simulink model "connecttoUDP_Testing"  (R2025a)
settings: Solver=ode4  StartTime=0.0  StopTime=inf  FixedStep=1/500  RelTol=1e-3  EnableMultiTasking=on
undefined symbols (not defined in the file): HIL, qc_get_step_size
libraries: quarc_library x10
settings Model: Creator=analu  LastModifiedBy=QARM4
settings SolverCC: PositivePriorityOrder=on
settings ModelReferenceCC: EnableRefExpFcnMdlSchedulingChecks=on
settings RTWCC: SystemTargetFile=quarc_win64.tlc  Toolchain=QUARC win64 | nmake (64-bit Windows)  BuildConfiguration=Faster Runs  Description=QUARC Win64 Target Using Toolchain
settings STFCustomTargetCC: SystemTargetFile=quarc_win64.tlc  TargetLangStandard=C99 (ISO)  MultiwordLength=2048.0  DynamicStringBufferSize=256.0  ConcurrentExecutionCompliant=on  UseToolchainInfoCompliant=on
settings GRTTargetCC: ExtMode=on  ExtModeMexFile=quarc_comm  ParMdlRefBuildCompliant=off  CompOptLevelCompliant=off  CombineOutputUpdateFcns=off  MatFileLogging=off  CPPClassGenCompliant=off  GRTInterface=on

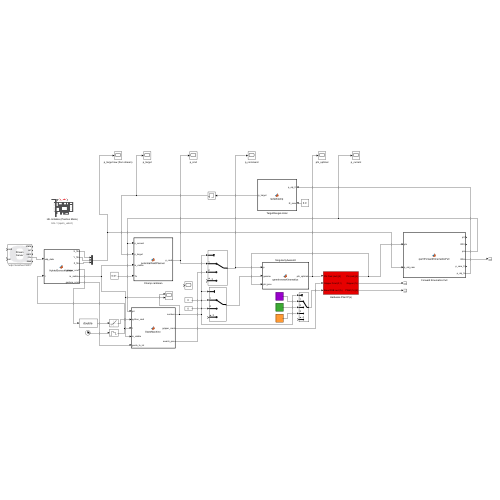
[thumbnail: Simulink's stored preview of the top-level diagram]
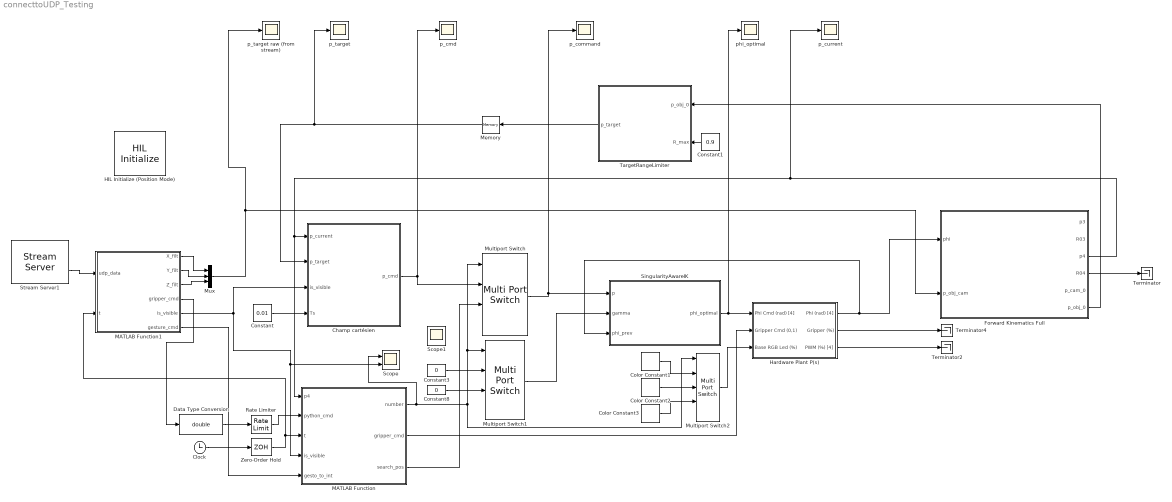
== system connecttoUDP_Testing ==
  Champ cartésien : MATLAB Function  TreatAsAtomicUnit=on
  Clock : Clock
  Color Constant1 : quarc_library/Sources/Signals/Color Constant  color=[0.6 0 0.8]
      settings: SourceProductName=QUARC Targets
  Color Constant2 : quarc_library/Sources/Signals/Color Constant  color=[0.23137 0.66667 0.19608]
      settings: SourceProductName=QUARC Targets
  Color Constant3 : quarc_library/Sources/Signals/Color Constant  color=[1 0.6 0.2]
      settings: SourceProductName=QUARC Targets
  Constant : Constant  Value=0.01
  Constant1 : Constant  Value=0.9
  Constant3 : Constant  Value=0
  Constant8 : Constant  Value=0
  Data Type Conversion : DataTypeConversion  OutMin=0  OutMax=11  OutDataTypeStr=double  SaturateOnIntegerOverflow=off  RndMeth=Floor
  Forward Kinematics Full : MATLAB Function  TreatAsAtomicUnit=on
  HIL Initialize (Position Mode) : quarc_library/Data Acquisition/Generic/Configuration/HIL Initialize  object_name=HIL-1  board_type=qarm_usb  board_number=0  board_options=j0_mode=0;j1_mode=0;j2_mode=0;j3_mode=0;gripper_mode=0;j0_profile_config=0;j0_profile_velocity=1.5708;j0_profile_acceleration=1.0472;j1_profile_config=0;j1_profile_velocity=1.5708;j1_profile_acceleration=1.0472;j2_profile_config=0;j2_profile_velocity=1.5708;j2_profile_acceleration=1.0472;j3_profile_config=0;j3_profile_velocity=1.5708;j3_profile_acceleration=1.0472;  exclusive=off  active=on  hardware_clocks=[0]  clock_modes=[]  initial_clock_frequencies=[]  set_clock_params_at_start=off  set_clock_params_at_switch_in=off  set_clock_frequencies_at_start=off  set_clock_frequencies_at_switch_in=off  analog_input_channels=[5:9]  analog_input_configurations=[]  analog_input_maximums=[]  analog_input_minimums=[]  set_analog_input_params_at_start=off  set_analog_input_params_at_switch_in=off  analog_output_channels=[]  analog_output_maximums=inf  analog_output_minimums=-inf  initial_analog_outputs=[0]  final_analog_outputs=[0]  watchdog_analog_outputs=[]  set_analog_output_params_at_start=off  set_analog_output_params_at_switch_in=off  set_analog_outputs_at_start=off  set_analog_outputs_at_switch_in=off  set_analog_outputs_at_terminate=off  set_analog_outputs_at_switch_out=off  set_analog_outputs_on_watchdog=off  digital_input_channels=[]  digital_output_channels=[]  digital_output_configuration=[]  initial_digital_outputs=[0]  final_digital_outputs=[0]  watchdog_digital_outputs=[0]  set_digital_output_params_at_start=off  set_digital_output_params_at_switch_in=off  set_digital_outputs_at_start=off  set_digital_outputs_at_switch_in=off  set_digital_outputs_at_terminate=off  set_digital_outputs_at_switch_out=off  set_digital_outputs_on_watchdog=off  encoder_channels=[]  quadrature=[]  encoder_filter_frequency=[]  initial_encoder_counts=[]  set_encoder_params_at_start=off  set_encoder_params_at_switch_in=off  set_encoder_counts_at_start=off  set_encoder_counts_at_switch_in=off  pwm_channels=[]  pwm_modes=[]  pwm_frequency=[]  pwm_configuration=[]  pwm_alignment=[]  pwm_polarity=[]  pwm_leading_deadband=[]  pwm_trailing_deadband=[]  initial_pwm_outputs=[]  final_pwm_outputs=[]  watchdog_pwm_outputs=[]  set_pwm_params_at_start=off  set_pwm_params_at_switch_in=off  set_pwm_outputs_at_start=off  set_pwm_outputs_at_switch_in=off  set_pwm_outputs_at_terminate=off  set_pwm_outputs_at_switch_out=off  set_pwm_outputs_on_watchdog=off  other_output_channels=[1000:1004 11000:11003 11005:11007]  initial_other_outputs=[zeros(1,9), ones(1,3)]  final_other_outputs=[zeros(1,9), ones(1,3)]  watchdog_other_outputs=zeros(1,12)  set_other_outputs_at_start=off  set_other_outputs_at_switch_in=off  set_other_outputs_at_terminate=on  set_other_outputs_at_switch_out=off  set_other_outputs_on_watchdog=off
  Hardware Plant P(s) : Subsystem
  MATLAB Function : MATLAB Function  TreatAsAtomicUnit=on
  MATLAB Function1 : MATLAB Function  TreatAsAtomicUnit=on
  Memory : Memory  InitialCondition=[0 ,0.5 ,0.5]
  Multiport Switch : MultiPortSwitch  SaturateOnIntegerOverflow=off  InputSameDT=off
  Multiport Switch1 : MultiPortSwitch  SaturateOnIntegerOverflow=off  InputSameDT=off
  Multiport Switch2 : MultiPortSwitch  Inputs=4  SaturateOnIntegerOverflow=off  InputSameDT=off
  Mux : Mux  Inputs=3
  Rate Limiter : RateLimiter  SampleTimeMode=inherited
  Scope : Scope  NumInputPorts=2
      settings: ActiveDisplayYMinimum=-0.24999999999999994  ActiveDisplayYMaximum=2.25  DataLoggingVariableName=ScopeData8
  Scope1 : Scope
      settings: DataLoggingVariableName=ScopeData9
  SingularityAwareIK : MATLAB Function  TreatAsAtomicUnit=on
  Stream Server1 : quarc_library/Communications/Basic/Stream Server  uri_source=Specify via dialog (do not evaluate)  uri=udp://localhost:5005  send_buffer_size=1460  receive_buffer_size=1460  byte_order=little endian (Intel - LSB first)  optimization=Minimum latency  send_options=Send all data  receive_options=Receive all data  default_value=[0,0,0,0,0,0,0,0]  sample_time=qc_get_step_size  active=off  implementation=Use blocking I/O in a separate thread  send_fifo_size=1000  receive_fifo_size=1000  send_priority=0  receive_priority=0  send_dimensions=off  receive_dimensions=off  max_dimensions=-1  data_type=single  type_expr=BusObject
      settings: AttributesFormatString="\"udp://localhost:5005\""
  TargetRangeLimiter : MATLAB Function  TreatAsAtomicUnit=on
  Terminator : Terminator
  Terminator2 : Terminator
  Terminator4 : Terminator
  Zero-Order Hold : ZeroOrderHold  SampleTime=-1
  p_cmd : Scope
      settings: ActiveDisplayYMinimum=-0.053062727209180587  ActiveDisplayYMaximum=0.31034032395109534
  p_command : Scope
      settings: ActiveDisplayYMinimum=-0.053062727209180587  ActiveDisplayYMaximum=0.31034032395109534  DataLoggingVariableName=ScopeData3
  p_current : Scope
      settings: ActiveDisplayYMinimum=-0.053062727209180587  ActiveDisplayYMaximum=0.31034032395109534  DataLoggingVariableName=ScopeData6
  p_target : Scope
      settings: ActiveDisplayYMinimum=-0.053062727209180587  ActiveDisplayYMaximum=0.31034032395109534  DataLoggingVariableName=ScopeData7
  p_target raw (from stream) : Scope
      settings: ActiveDisplayYMinimum=-0.053062727209180587  ActiveDisplayYMaximum=0.31034032395109534  DataLoggingVariableName=ScopeData2
  phi_optimal : Scope
      settings: ActiveDisplayYMinimum=-0.053062727209180587  ActiveDisplayYMaximum=0.31034032395109534
  wires:
  Stream Server1/4 -> MATLAB Function1/1(udp_data)
  SingularityAwareIK/1(phi_optimal) -> phi_optimal/1, Hardware Plant P(s)/1(Phi Cmd (rad) [4])
  Constant/1 -> Champ cartésien/4(Ts)
  Hardware Plant P(s)/1(Phi (rad) [4]) -> SingularityAwareIK/3(phi_prev), Forward Kinematics Full/1(phi)
  Hardware Plant P(s)/2(Gripper (%)) -> Terminator4/1
  Hardware Plant P(s)/3(PWM (%) [4]) -> Terminator2/1
  Multiport Switch/1 -> p_command/1, SingularityAwareIK/1(p)
  Champ cartésien/1(p_cmd) -> p_cmd/1, Multiport Switch/2
  MATLAB Function/3(search_pos) -> Multiport Switch/3
  MATLAB Function/2(gripper_cmd) -> Hardware Plant P(s)/2(Gripper Cmd (0,1))
  Multiport Switch2/1 -> Hardware Plant P(s)/3(Base RGB Led (%))
  Multiport Switch1/1 -> SingularityAwareIK/2(gamma)
  MATLAB Function/1(number) -> Scope/1, Multiport Switch2/1, Multiport Switch/1, Multiport Switch1/1
  Constant3/1 -> Multiport Switch1/2
  Constant8/1 -> Multiport Switch1/3
  Zero-Order Hold/1 -> MATLAB Function1/2(t), MATLAB Function/3(t)
  Clock/1 -> Zero-Order Hold/1
  Rate Limiter/1 -> MATLAB Function/2(python_cmd)
  Data Type Conversion/1 -> Rate Limiter/1
  Forward Kinematics Full/3(p4) -> p_current/1, MATLAB Function/1(p4), Champ cartésien/1(p_current)
  Forward Kinematics Full/4(R04) -> Terminator/1
  Forward Kinematics Full/6(p_obj_0) -> TargetRangeLimiter/1(p_obj_0)
  TargetRangeLimiter/1(p_target) -> Memory/1
  Color Constant2/1 -> Multiport Switch2/3
  Color Constant1/1 -> Multiport Switch2/2
  Color Constant3/1 -> Multiport Switch2/4
  Constant1/1 -> TargetRangeLimiter/2(R_max)
  Memory/1 -> p_target/1, Champ cartésien/2(p_target)
  MATLAB Function1/5(is_visible) -> Scope/2, MATLAB Function/4(is_visible), Champ cartésien/3(is_visible)
  Mux/1 -> p_target raw (from stream)/1, Forward Kinematics Full/2(p_obj_cam)
  MATLAB Function1/1(X_filt) -> Mux/1
  MATLAB Function1/2(Y_filt) -> Mux/2
  MATLAB Function1/3(Z_filt) -> Mux/3
  MATLAB Function1/4(gripper_cmd) -> Data Type Conversion/1
  MATLAB Function1/6(gesture_cmd) -> MATLAB Function/5(gesto_to_int)

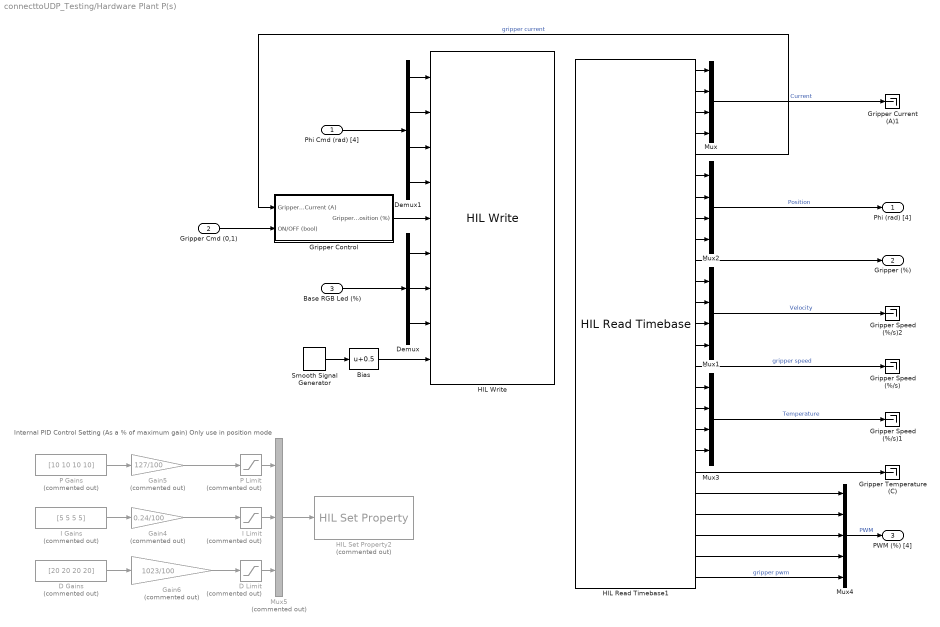
== system connecttoUDP_Testing/Hardware Plant P(s) ==
  note: Internal PID Control Setting (As a % of maximum gain)
      | Only use in position mode
  Phi Cmd (rad) [4] : Inport
  Gripper Cmd (0,1) : Inport  Port=2
  Base RGB Led (%) : Inport  Port=3
  Bias : Bias  Bias=0.5  SaturateOnIntegerOverflow=off
  D Gains : Constant  Commented=on  Value=[20 20 20 20]
  D Limit : Saturate  Commented=on  UpperLimit=[1023 1023 1023 1023]  LowerLimit=[0 0 0 0]
  Demux : Demux  Outputs=3
  Demux1 : Demux
  Gain4 : Gain  Commented=on  Gain=0.24/100
  Gain5 : Gain  Commented=on  Gain=127/100
  Gain6 : Gain  Commented=on  Gain=1023/100
  Gripper Control : Subsystem
  Gripper Current (A)1 : Terminator
  Gripper Speed (%/s) : Terminator
  Gripper Speed (%/s)1 : Terminator
  Gripper Speed (%/s)2 : Terminator
  Gripper Temperature (C) : Terminator
  HIL Read Timebase1 : quarc_library/Data Acquisition/Generic/Timebases/HIL Read Timebase  object_name=HIL-1  clock=0  analog_channels=[5:9]  encoder_channels=[]  digital_channels=[]  other_channels=[1000:1004 3000:3004 10000:10004 11000:11004]  active=on  vector_output=off  data_type_mode=Inherit via back propagation  encoder_data_type=double  digital_data_type=boolean  overflow_mode=Error on overflow  samples_in_buffer=max(ceil(1/qc_get_step_size), 1)
  HIL Set Property2 : quarc_library/Data Acquisition/Generic/Configuration/HIL Set Property  Commented=on  object_name=unassigned  property_type=2  property_codes=[128:131 133:136 138:141]  property_source=2  property_value_num=0  set_at_start=on  sample_time=-1  active=off
      settings: AttributesFormatString=(%<object_name>)  SourceProductName=QUARC Targets
  HIL Write : quarc_library/Data Acquisition/Generic/Immediate I//O/HIL Write  object_name=HIL-1  analog_channels=[]  pwm_channels=[]  digital_channels=[]  other_channels=[1000:1004 11005:11008]  sample_time=-1  active=on  vector_input=off
  I Gains : Constant  Commented=on  Value=[5 5 5 5]
  I Limit : Saturate  Commented=on  UpperLimit=[0.24 0.24 0.24 0.24]  LowerLimit=[0 0 0 0]
  Mux{,1..3} (4 alike) : Mux
  Mux4 : Mux  Inputs=5
  Mux5 : Mux  Commented=on  Inputs=3
  P Gains : Constant  Commented=on  Value=[10 10 10 10]
  P Limit : Saturate  Commented=on  UpperLimit=[127 127 127 127]  LowerLimit=[0 0 0 0]
  Smooth Signal Generator : quarc_library/Sources/Signals/Smooth Signal Generator  signal_type=Sine  source=Internal (dialog parameters)  amplitude=0.5  frequency=60/72  initial_phase=0  sample_time=qc_get_step_size  output_cos=off
      settings: SourceProductName=QUARC Targets
  Phi (rad) [4] : Outport  VectorParamsAs1DForOutWhenUnconnected=off
  Gripper (%) : Outport  Port=2  VectorParamsAs1DForOutWhenUnconnected=off
  PWM (%) [4] : Outport  Port=3  VectorParamsAs1DForOutWhenUnconnected=off
  wires:
  HIL Read Timebase1/10 -> Gripper (%)/1
  Mux4/1 -> PWM (%) [4]/1  "PWM"
  HIL Read Timebase1/25 -> Mux4/5  "gripper pwm"
  HIL Read Timebase1/24 -> Mux4/4
  HIL Read Timebase1/23 -> Mux4/3
  HIL Read Timebase1/22 -> Mux4/2
  HIL Read Timebase1/21 -> Mux4/1
  Mux2/1 -> Phi (rad) [4]/1  "Position"
  Phi Cmd (rad) [4]/1 -> Demux1/1
  Demux1/4 -> HIL Write/4
  Demux1/3 -> HIL Write/3
  Demux1/2 -> HIL Write/2
  Demux1/1 -> HIL Write/1
  Base RGB Led (%)/1 -> Demux/1
  Mux3/1 -> Gripper Speed (%/s)1/1  "Temperature"
  Mux1/1 -> Gripper Speed (%/s)2/1  "Velocity"
  Mux/1 -> Gripper Current (A)1/1  "Current"
  HIL Read Timebase1/20 -> Gripper Temperature (C)/1
  HIL Read Timebase1/1 -> Mux/1
  HIL Read Timebase1/2 -> Mux/2
  HIL Read Timebase1/13 -> Mux1/3
  Demux/2 -> HIL Write/7
  HIL Read Timebase1/19 -> Mux3/4
  Demux/1 -> HIL Write/6
  HIL Read Timebase1/11 -> Mux1/1
  HIL Read Timebase1/16 -> Mux3/1
  HIL Read Timebase1/17 -> Mux3/2
  HIL Read Timebase1/3 -> Mux/3
  Demux/3 -> HIL Write/8
  HIL Read Timebase1/15 -> Gripper Speed (%/s)/1  "gripper speed"
  HIL Read Timebase1/5 -> Gripper Control/1(Gripper Current (A))  "gripper current"
  HIL Read Timebase1/7 -> Mux2/2
  HIL Read Timebase1/4 -> Mux/4
  HIL Read Timebase1/12 -> Mux1/2
  HIL Read Timebase1/8 -> Mux2/3
  HIL Read Timebase1/18 -> Mux3/3
  HIL Read Timebase1/6 -> Mux2/1
  HIL Read Timebase1/9 -> Mux2/4
  HIL Read Timebase1/14 -> Mux1/4
  Gripper Control/1(Gripper Position (%)) -> HIL Write/5
  Gripper Cmd (0,1)/1 -> Gripper Control/2(ON/OFF (bool))
  Smooth Signal Generator/1 -> Bias/1
  Bias/1 -> HIL Write/9
  I Limit/1 -> Mux5/2
  Gain5/1 -> P Limit/1
  D Limit/1 -> Mux5/3
  Mux5/1 -> HIL Set Property2/1
  I Gains/1 -> Gain4/1
  P Gains/1 -> Gain5/1
  D Gains/1 -> Gain6/1
  P Limit/1 -> Mux5/1
  Gain6/1 -> D Limit/1
  Gain4/1 -> I Limit/1

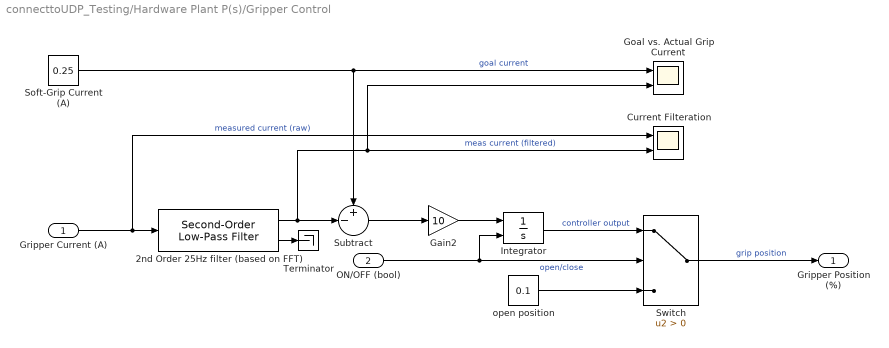
== system connecttoUDP_Testing/Hardware Plant P(s)/Gripper Control ==
  Gripper Current (A) : Inport
  ON/OFF (bool) : Inport  Port=2
  2nd Order 25Hz filter (based on FFT) : quarc_library/Continuous/Second-Order Low-Pass Filter  params_source=Internal (dialog parameters)  input_width=25*2*pi  input_zeta=1  input_init=0
  Current Filteration : Scope  NumInputPorts=2
      settings: ActiveDisplayYMinimum=-0.01447  ActiveDisplayYMaximum=0.62651  DataLoggingVariableName=ScopeData5
  Gain2 : Gain  Gain=10
  Goal vs. Actual Grip Current : Scope  NumInputPorts=2
      settings: ActiveDisplayYMinimum=0.00229  ActiveDisplayYMaximum=0.27702  DataLoggingVariableName=ScopeData4
  Integrator : Integrator  ExternalReset=either  InitialCondition=0.1  LimitOutput=on  UpperSaturationLimit=0.9  LowerSaturationLimit=0.1
  Soft-Grip Current (A) : Constant  Value=0.25
  Subtract : Sum  Inputs=+-|
  Switch : Switch  Criteria=u2 > Threshold  SaturateOnIntegerOverflow=off  InputSameDT=off
  Terminator : Terminator
  open position : Constant  Value=0.1
  Gripper Position (%) : Outport  VectorParamsAs1DForOutWhenUnconnected=off
  wires:
  Gripper Current (A)/1 -> 2nd Order 25Hz filter (based on FFT)/1, Current Filteration/1  "measured current (raw)"
  ON/OFF (bool)/1 -> Switch/2, Integrator/2  "open/close"
  open position/1 -> Switch/3
  Switch/1 -> Gripper Position (%)/1  "grip position"
  Soft-Grip Current (A)/1 -> Subtract/1, Goal vs. Actual Grip Current/1  "goal current"
  2nd Order 25Hz filter (based on FFT)/1 -> Subtract/2, Current Filteration/2, Goal vs. Actual Grip Current/2  "meas current (filtered)"
  Subtract/1 -> Gain2/1
  Integrator/1 -> Switch/1  "controller output"
  Gain2/1 -> Integrator/1
  2nd Order 25Hz filter (based on FFT)/2 -> Terminator/1

== matlab function connecttoUDP_Testing/TargetRangeLimiter ==
  data: p_obj_0 input size=3; p_target output size=3; R_max input
function p_target = radialClamp(p_obj_0, R_max)

eps_val = 1e-6;

norm_p = norm(p_obj_0);

if norm_p > R_max
    p_target = R_max * (p_obj_0 / (norm_p + eps_val));
else
    p_target = p_obj_0;
end

end

== matlab function connecttoUDP_Testing/Champ cartésien ==
  data: p_current input; p_cmd output; p_target input; is_visible input; Ts input
function p_cmd = potentialFieldPlanner(p_current, p_target, is_visible, Ts)
% p_current : [3x1]
% p_target   : [3x1]
% is_visible: 0/1
% Ts        : pas de temps

%% Paramètres
k_att = 2.0;       % gain attractif
k_rep = 0.05;      % gain répulsif cylindre
v_max = 0.25;      % vitesse cartésienne max [m/s]

d0 = 0.15;         % rayon d'influence du cylindre
eps_norm = 1e-6;   % protection division par zéro

%% Si cible non visible : on garde la position actuelle
if is_visible == 0
    p_cmd = p_current;
    return;
end

%% --- Champ attractif ---
e = p_target - p_current;
F_att = k_att * e;

%% --- Champ répulsif cylindre autour de la base ---
x = p_current(1);
y = p_current(2);
d = sqrt(x^2 + y^2);

F_rep = [0;0;0];

if d < d0 && d > eps_norm
    n = [x; y; 0] / (d + eps_norm);
    F_rep = k_rep * (1/d - 1/d0) * (1/(d^2 + eps_norm)) * n;
end

%% --- Champ total ---
F = F_att + F_rep;

%% --- Saturation smooth ---
F_norm = norm(F);

if F_norm > eps_norm
    v_cmd = v_max * tanh(F_norm / v_max) * (F / F_norm);
else
    v_cmd = [0;0;0];
end

%% --- Pas d'Euler ---
p_cmd = p_current + Ts * v_cmd;

end

== matlab function connecttoUDP_Testing/Forward Kinematics Full ==
  data: p3 output; R03 output; phi input; p4 output; R04 output; p_obj_cam input; p_cam_0 output; p_obj_0 output
function [p3, R03, p4, R04, p_cam_0, p_obj_0] = qarmForwardKinematicsFull(phi, p_obj_cam)
%% QARM Forward Kinematics Full
% INPUTS:
%   phi       : angles articulaires QArm [4x1]
%   p_obj_cam : position objet dans le repère caméra [3x1]
%               (mettre [0;0;0] si non utilisée)
%
% OUTPUTS:
%   p3      : position frame {3} dans {0}
%   R03     : rotation frame {3} dans {0}
%   p4      : position effecteur frame {4} dans {0}
%   R04     : rotation effecteur frame {4} dans {0}
%   p_cam_0 : position caméra dans {0}
%   p_obj_0 : position objet dans {0}

%% Paramètres du manipulateur
L1 = 0.1400;
L2 = 0.3500;
L3 = 0.0500;
L4 = 0.2500;
L5 = 0.1500;

%% Paramètres alternatifs
l1 = L1;
l2 = sqrt(L2^2 + L3^2);
l3 = L4 + L5;
beta = atan(L3/L2);

%% Conversion phi -> theta
theta = phi;
theta(1) = phi(1);
theta(2) = phi(2) + beta - pi/2;
theta(3) = phi(3) - beta;
theta(4) = phi(4);

%% Matrices homogènes
T01 = quanser_arm_DH(  0, -pi/2, l1, theta(1) );
T12 = quanser_arm_DH( l2,     0,  0, theta(2) );
T23 = quanser_arm_DH(  0, -pi/2,  0, theta(3) );
T34 = quanser_arm_DH(  0,     0, l3, theta(4) );

T02 = T01*T12;
T03 = T02*T23;
T04 = T03*T34;

%% Sorties principales
p3  = T03(1:3,4);
R03 = T03(1:3,1:3);

p4  = T04(1:3,4);
R04 = T04(1:3,1:3);

%% Caméra
d_tilde = 0.3;                 % distance entre P03 et la caméra
p_cam_3 = [0;0;d_tilde];

% Choisir UNE SEULE orientation caméra
R_cam_3 = [ 0 -1  0;
            1  0  0;
            0  0  1 ];

p_cam_0 = p3 + R03 * p_cam_3;
R_cam_0 = R03 * R_cam_3;

%% Objet
if nargin < 2
    p_obj_cam = [0;0;0];
end

p_obj_0 = p_cam_0 + R_cam_0 * p_obj_cam;

end

function T = quanser_arm_DH(a, alpha, d, theta)

T_R_z = [cos(theta) -sin(theta) 0 0;
         sin(theta)  cos(theta) 0 0;
                  0           0 1 0;
                  0           0 0 1];

T_T_z = [1 0 0 0;
         0 1 0 0;
         0 0 1 d;
         0 0 0 1];

T_T_x = [1 0 0 a;
         0 1 0 0;
         0 0 1 0;
         0 0 0 1];

T_R_x = [1          0           0 0;
         0 cos(alpha) -sin(alpha) 0;
         0 sin(alpha)  cos(alpha) 0;
         0          0           0 1];

T = T_R_z * T_T_z * T_T_x * T_R_x;

end

== matlab function connecttoUDP_Testing/SingularityAwareIK ==
  data: p input; gamma input; phi_optimal output; phi_prev input
function phi_optimal = qarmInverseKinematics(p, gamma, phi_prev)
%% QARM Inverse Kinematics with singularity avoidance
% Gère :
% 1) singularité "effecteur au-dessus de la base" via exclusion cylindrique
% 2) singularité de l'articulation 3 : theta3 = +/- 90 deg
%
% INPUTS:
%   p        : position [x;y;z] en m
%   gamma    : rotation poignet (rad)
%   phi_prev : configuration précédente [4x1] en rad
%
% OUTPUT:
%   phi_optimal : configuration atteignable [4x1] rad

%% Paramètres du manipulateur
L1 = 0.1400; 
L2 = 0.3500; 
L3 = 0.0500; 
L4 = 0.2500; 
L5 = 0.1500;

beta = atan(L3/L2);

lambda1 = L1;
lambda2 = sqrt(L2^2 + L3^2);
lambda3 = L4 + L5;

%% Paramètres d'évitement des singularités A ADAPTER PAS ENCORE DE TEST FAIT SUR ROBOT 
R_MIN = 0.08;                 % rayon mini du cylindre d'exclusion (m)
EPS_DEN = 1e-6;               % protection divisions
EPS_COST = 1e-4;              % protection coût singularité

W_CONT = 1.0;                 % poids continuité avec phi_prev
W_SING_THETA3 = 0.25;         % poids singularité theta3 = +/- pi/2
W_LIMIT = 0.05;               % petit poids pour éloigner des butées

%% --- 1) Exclusion cylindrique autour de la base ---
% On évite une zone cylindrique autour de la base (le bras se bloque quand
% il y entre).
% Ici, on régularise directement la cible cartésienne.
p_reg = p;
r = hypot(p(1), p(2));

if r < R_MIN
    if r > EPS_DEN
        p_reg(1) = p(1) * R_MIN / r;
        p_reg(2) = p(2) * R_MIN / r;
    else
        % Si on est exactement sur l'axe, on prend la direction de la base précédente
        base_dir = phi_prev(1);
        p_reg(1) = R_MIN * cos(base_dir);
        p_reg(2) = R_MIN * sin(base_dir);
    end
end

%% Initialisation
theta = zeros(4,4);
phi   = zeros(4,4);

%% --- Calcul theta2 / theta3 ---
A = lambda2; 
C = -lambda3; 
H = lambda1 - p_reg(3);

D1 = -hypot(p_reg(1), p_reg(2)); 
D2 =  hypot(p_reg(1), p_reg(2));

F1 = (D1^2 + H^2 - A^2 - C^2)/(2*A);
F2 = (D2^2 + H^2 - A^2 - C^2)/(2*A);

% Si racine négative, saturation
if C^2 - F1^2 < 0
    warning('Position non atteignable pour solution 1/2 : saturation');
    theta(3,1) = sign(C)*pi/2;
    theta(3,2) = sign(C)*pi/2;
else
    theta(3,1) = 2*atan2(C + sqrt(C^2 - F1^2), F1);
    theta(3,2) = 2*atan2(C - sqrt(C^2 - F1^2), F1);
end

if C^2 - F2^2 < 0
    warning('Position non atteignable pour solution 3/4 : saturation');
    theta(3,3) = sign(C)*pi/2;
    theta(3,4) = sign(C)*pi/2;
else
    theta(3,3) = 2*atan2(C + sqrt(C^2 - F2^2), F2);
    theta(3,4) = 2*atan2(C - sqrt(C^2 - F2^2), F2);
end

%% --- Calcul theta2 ---
for i = 1:4
    D = D1; 
    if i > 2
        D = D2; 
    end

    M = A + C*sin(theta(3,i));
    N = -C*cos(theta(3,i));

    if abs(M) < EPS_DEN
        M = sign_nonzero(M) * EPS_DEN;
    end

    cos_term = (D*M + H*N)/(M^2 + N^2);
    sin_term = (H - N*cos_term)/M;
    theta(2,i) = atan2(sin_term, cos_term);
end

%% --- Calcul theta1 ---
for i = 1:4
    denom = lambda2*cos(theta(2,i)) - lambda3*sin(theta(2,i)+theta(3,i));
    if abs(denom) < EPS_DEN
        denom = sign_nonzero(denom) * EPS_DEN;
    end
    theta(1,i) = atan2(p_reg(2)/denom, p_reg(1)/denom);
end

%% --- Remap vers angles QARM ---
phi(1,:) = theta(1,:);
phi(2,:) = theta(2,:) - beta + pi/2;
phi(3,:) = theta(3,:) + beta;
phi(4,:) = gamma;

phi = wrapToPiLocal(phi);

%% --- Saturation des limites ---
for i = 1:4
    phi(:,i) = saturate_joint_limits(phi(:,i));
end

%% --- Choix de la meilleure solution avec pénalisation singularités ---
phi_optimal = phi(:,1);
best_cost = candidate_cost(phi(:,1), theta(:,1), phi_prev, R_MIN, r, W_CONT, W_SING_THETA3, W_LIMIT, EPS_COST);

for i = 2:4
    current_cost = candidate_cost(phi(:,i), theta(:,i), phi_prev, R_MIN, r, W_CONT, W_SING_THETA3, W_LIMIT, EPS_COST);
    if isnan(current_cost)
        continue;
    end
    if current_cost < best_cost
        phi_optimal = phi(:,i);
        best_cost = current_cost;
    end
end

if any(isnan(phi_optimal))
    warning('NaN détecté dans phi_optimal, retour à phi_prev');
    phi_optimal = phi_prev;
end

end

%% ===================== COST FUNCTION =====================
function J = candidate_cost(phi_i, theta_i, phi_prev, R_MIN, r_raw, W_CONT, W_SING_THETA3, W_LIMIT, EPS_COST)

    % 1) Continuité avec la configuration précédente
    dphi = wrapToPiLocal(phi_i - phi_prev);
    J_cont = norm(dphi);

    % 2) Pénalisation singularité theta3 = +/- 90 deg
    % Rapport : singularité quand theta3 = +/- pi/2
    d1 = abs(wrapToPiLocal(theta_i(3) - pi/2));
    d2 = abs(wrapToPiLocal(theta_i(3) + pi/2));
    J_sing_theta3 = 1/(d1^2 + EPS_COST) + 1/(d2^2 + EPS_COST);

    % 3) Petite pénalisation si on est près des butées
    J_limits = joint_limit_barrier(phi_i, EPS_COST);

    % 4) Pénalisation brute si la cible originale était trop près de l'axe base
    % (même si régularisée ensuite)
    if r_raw < R_MIN
        J_base = 1 + 10*(R_MIN - r_raw)^2;
    else
        J_base = 0;
    end

    J = W_CONT * J_cont + ...
        W_SING_THETA3 * J_sing_theta3 + ...
        W_LIMIT * J_limits + ...
        J_base;
end

%% ===================== JOINT LIMITS =====================
function phi_sat = saturate_joint_limits(phi)
% C'est les mêmes limites qu'avant mais ça peut être intéressant à régler 
limits = [
    -170  170;
    -80    80;
    -95    75;
    -160  160
] * pi/180;

phi_sat = phi;
for i = 1:4
    if phi(i) < limits(i,1)
        phi_sat(i) = limits(i,1);
    end
    if phi(i) > limits(i,2)
        phi_sat(i) = limits(i,2);
    end
end
end

function J = joint_limit_barrier(phi, eps_cost)
limits = [
    -170  170;
    -80    80;
    -95    75;
    -160  160
] * pi/180;

J = 0;
for k = 1:4
    dmin = abs(phi(k) - limits(k,1));
    dmax = abs(limits(k,2) - phi(k));
    J = J + 1/(dmin^2 + eps_cost) + 1/(dmax^2 + eps_cost);
end
end

%% ===================== HELPERS =====================
function y = wrapToPiLocal(x)
y = mod(x + pi, 2*pi) - pi;
end

function s = sign_nonzero(x)
if x >= 0
    s = 1;
else
    s = -1;
end
end

== matlab function connecttoUDP_Testing/MATLAB Function1 ==
  data: udp_data input size=[8 1]; X_filt output; t input size=1; Y_filt output; Z_filt output; gripper_cmd output; is_visible output; gesture_cmd output size=1
function [X_filt, Y_filt, Z_filt, gripper_cmd, is_visible, gesture_cmd] = HybridSensorKalman(udp_data, t)
    % udp_data is a 7x1 vector from Python: 
    % [SensX, SensY, SensZ, PinhX, PinhY, PinhZ, FoundFlag]
    
    % Define the variables that will remember their values between Simulink steps
    persistent x_est P kf_initialized t_grip_start

    % Initialize the Kalman Filter
    if isempty(kf_initialized)
        x_est = [0.2; 0.0; 0.3]; % Initial guess (Safe home position)
        P = eye(3) * 1.0;        % Initial uncertainty
        kf_initialized = true;
        t_grip_start = -1;       % Timer for gripper delay
    end

    % 1. Unpack UDP data and force double precision
    z_sens = double(udp_data(1:3));
    z_pinh = double(udp_data(4:6));
    found_flag = double(udp_data(7));
    gesture_cmd = double(udp_data(8));

    is_visible = found_flag;
    
    % Kalman tuning parameters (to be adjusted through trial and error)
    Q = eye(3) * 0.001; % Process Noise
    R_val = 0.05;       % Measurement Noise

    % 2. Constant Position Kalman Prediction
    x_est = x_est; 
    P = P + Q;

    % 3. Kalman Update (Sensor Fusion)
    if found_flag == 1
        % Determine depth
        depth = z_sens(3);
        if depth == 0 % Blind sensor scenario
            depth = z_pinh(3);
        end
        
        % Dynamic Confidence (Soft Switch)
        if depth < 0.25
            % Very close: Trust Pinhole 100%, Sensor 0%
            w_sens = 0.0; 
            w_pinh = 1.0;
        elseif depth > 0.35
            % Far away: Trust Sensor 100%, Pinhole 0%
            w_sens = 1.0; 
            w_pinh = 0.0;
        else
            % Transition Zone (25cm to 35cm): Cross-fade the signals
            w_sens = (depth - 0.25) / 0.10; 
            w_pinh = 1.0 - w_sens;
        end
        
        % Fused depth estimation
        z_fused = (w_sens * z_sens) + (w_pinh * z_pinh);
        
        % Calculate Kalman Gain
        R = eye(3) * R_val;
        K = P / (P + R);
        
        % Apply the measurement correction
        x_est = x_est + K * (z_fused - x_est);
        P = (eye(3) - K) * P;
    end

    % 4. Output filtered coordinates
    X_filt = x_est(1);
    Y_filt = x_est(2);
    Z_filt = x_est(3);

    % 5. Gripper Delay Logic
    gripper_cmd = 0;
    
    % Calculate distance from arm base (assuming base is 0,0,0)
    dist_to_target = norm(x_est); 

    if found_flag == 1 && dist_to_target <= 0.18 % COMMIT_DISTANCE variable
        if t_grip_start == -1
            t_grip_start = t; % Start timer
        elseif (t - t_grip_start) >= 0.75 % GRIP_DELAY variable
            gripper_cmd = 1; % Trigger grip
        end
    else
        t_grip_start = -1; % Reset timer if it moves away
    end
end

== matlab function connecttoUDP_Testing/MATLAB Function ==
  data: number output; p4 input; python_cmd input; t input; is_visible input; gripper_cmd output; search_pos output; gesto_to_int input
function [number, gripper_cmd, search_pos] = StateMachine(p4, python_cmd, t, is_visible, gesto_to_int)    
    
    persistent state
    persistent t_travel
    persistent t_visible
    persistent t_lost
    persistent t_gesture
    persistent current_y

    if isempty(state)
        state = 2; % 0 = Hunting the ball down, 1 = Going back to goal, 2 = Returning home and search
        t_travel = -1; % Putting a negative time stops the timer, used to find the travel time in each state mode
        t_visible = -1;
        t_lost = -1;
        t_gesture = -1;
        current_y = 0;
    end
    
    % Default safe position to output when not in State 2
    search_pos = [0.25; 0; 0.50];

    % --- Machine State Logic ---
    switch state
        
        case 0 % STATE 0: HUNTING THE BALL
            number = 1; % Connected on port 1 (xyz_mean)
            gripper_cmd = python_cmd; % The claw follows the camera
            
            % 1. CHECK IF BALL WAS CAUGHT
            if python_cmd == 1
                state = 3; 
                t_lost = -1; % Reset lost timer just in case
            end
            
            % 2. WATCHDOG TIMER: IF BALL IS LOST
            % If the camera goes blind, start the stopwatch before aborting
            if is_visible == 0
                if t_lost == -1
                    t_lost = t; % Start the lost stopwatch
                elseif (t - t_lost) >= 2.5 % Lost for more than 2.5 seconds
                    state = 2; % Go back to search mode
                    t_lost = -1; % Reset timer
                end
            else
                % Ball is visible, reset the stopwatch (Debounce)
                t_lost = -1; 
            end
            
        case 1 % STATE 1: DELIVERY (Advance in a straight line and release)
            number = 2; % We use port 2 to send a dynamic search_pos
            
            % 1. CALCULATE THE DYNAMIC TARGET POSITION
            % X was 0.25. We scale it by 2.25
            % Y is scaled by 2.25 in the exact same direction
            % Z is lowered to 0.40m
            target_x = 0.25 * 2.25; 
            target_y = current_y * 2.25;
            target_pos = [target_x; target_y; 0.40];
            
            % Send this position to the kinematics
            search_pos = target_pos; 
            
            % 2. IDENTIFY ARRIVAL AT TARGET
            distance_goal = norm(p4(1:3) - target_pos);
            
            if distance_goal < 0.05 && t_travel == -1
                t_travel = t; % Arrived! Start the delivery stopwatch  
            end
            
            % 3. DELIVERY TIMER LOGIC (Wait 3s -> Drop -> Wait 1s -> Leave)
            if t_travel ~= -1
                % If 4 seconds have passed (3s holding + 1s letting go)
                if (t - t_travel) >= 4.0
                    state = 2; % Mission accomplished! Return to Home/Search
                    t_travel = -1; % Reset timer
                    current_y = 0; % Reset joystick memory for next time
                    gripper_cmd = 1; % Claw still closed
                    
                % If 3 seconds have passed
                elseif (t - t_travel) >= 3.0 
                    gripper_cmd = 0; % OPEN CLAW (Drop the ball)
                    
                % If arrived but still waiting the initial 3 seconds
                else
                    gripper_cmd = 1; % KEEP CLAW CLOSED
                end
                
            else
                % Still traveling to the target
                gripper_cmd = 1; % Keep holding the ball tight
            end

        case 2 % STATE 2: SEARCH MODE (Go to alert position and sweep)
            number = 2; % Connected on port 2 (Search position)
            gripper_cmd = 0; % Keep claw open to not grab ghosts
            
            % 1. IDENTIFY ARRIVAL AT ALERT POSITION (Home)
            % Calculates distance to the base center position [0.25; 0; 0.50]
            distance_home = norm(p4(1:3) - [0.25; 0; 0.50]); 
            
            if distance_home < 0.05 && t_travel == -1
                t_travel = t; 
            end
            
            % 2. EXECUTE THE SINE WAVE SWEEP
            if t_travel == -1
                % Not there yet, keep target strictly at the center
                search_pos = [0.25; 0; 0.50];
            else
                % Start oscillating the Y axis                
                y_sweep = 0.25 * sin(0.30 * (t - t_travel));
                search_pos = [0.25; y_sweep; 0.50];
            end
            
            % 3. VERIFICATION BARRIER (DEBOUNCE LOGIC)
            if is_visible == 1
                if t_visible == -1
                    t_visible = t; % Ball spotted, start the stopwatch
                elseif (t - t_visible) >= 0.25 % Has it been consistently visible for 0.25 second
                    state = 3; % Barrier cleared! Transition to HUNTING
                    t_travel = -1; % Reset sweep timer
                    t_visible = -1; % Reset vision timer
                end
            else
                % False alarm or lost sight --> Reset stopwatch immediately
                t_visible = -1;
            end             

        case 3 % STATE 3: HOLD TARGET AND GESTURE JOYSTICK CONTROL
            number = 2; % Connect on port 2 (Search/Home position)
            gripper_cmd = 1; % KEEP CLAW CLOSED (Holding the ball)
            
            % 1. IDENTIFY ARRIVAL AT ALERT POSITION (Home)
            % Calculates distance to the base center position [0.25; 0; 0.50]
            distance_home = norm(p4(1:3) - [0.25; 0; 0.50]); 
            
            if distance_home < 0.05 && t_travel == -1
                t_travel = t; % Arrived! Unlock joystick control
                current_y = 0; % Reset joystick position to absolute center
            end
            
            % 2. EXECUTE THE JOYSTICK MOVEMENT BASED ON GESTURE
            if t_travel == -1
                % Not there yet, keep target strictly at the center
                search_pos = [0.25; 0; 0.50];
            else
                % Arrived at center. Now read the gesture to move!
                if gesto_to_int == 3 % RIGHT
                    current_y = current_y + 0.00005; % Move right smoothly
                    
                elseif gesto_to_int == 4 % LEFT
                    current_y = current_y - 0.00005; % Move left smoothly
                    
                end
                % Note: If gesture is NONE (0) or HAND (2), current_y is NOT modified. 
                % This creates the "freeze in place" smooth stop effect!
                
                % 3. SAFETY CLAMP (Mechanical Limits)
                % Prevent the arm from rotating beyond safe boundaries
                if current_y > 0.25
                    current_y = 0.25;
                elseif current_y < -0.25
                    current_y = -0.25;
                end
                
                % Output the accumulated position to the kinematics
                search_pos = [0.25; current_y; 0.50];
            end
            
            % 4. STOP GESTURE AND TRANSITION (With Debounce/Safety)
            % If the stop sign is shown AND the robot is already parked
            if gesto_to_int == 1 && t_travel ~= -1
                if t_gesture == -1
                    t_gesture = t; % AI saw STOP! Start the stopwatch
                elseif (t - t_gesture) >= 0.5 % Has it been a STOP for 0.5s?
                    state = 1; % Transition to the DELIVERY state
                    t_travel = -1; % Reset timer for the next state
                    t_gesture = -1; % Reset gesture timer
                end
            else
                % If it's not a STOP sign (false alarm or still moving), reset stopwatch
                t_gesture = -1; 
            end
            
        otherwise
            % Security against bugs 

            % 1. Fallback to the safest physical state
            state = 2; 
            number = 2; 
            search_pos = [0.25; 0; 0.50]; 
            gripper_cmd = 0; 
            
            % 2. Wipe all memory clean (Reset all timers)
            t_travel = -1;
            t_visible = -1;
            t_lost = -1;
            t_gesture = -1;
            current_y = 0;
    end
end
